simulink model "procestest"  (R2022b)
settings: Solver=VariableStepAuto  StartTime=0.0  StopTime=10.0  RelTol=1e-3
values from neighbouring files (symbols this model uses):
  A = 1/(4*tita*tita*sqrt(2))    [controllerId.m]    (also in identif_tf.m = 0.00679290871522)
  Cd = 1    [identif_tf.m]
  g = 9.8    [identif_tf.m]
  m = 2.7/1000    (= 0.0027)    [identif_tf.m]
  pwm_values = [0 20 60 100]    [identif_tf.m]
  q_points = [0 0.5 1.3 1.55]    [identif_tf.m]
  ro = 1.225    [identif_tf.m]
  Vb = (4*pi*(d_ball/2)^3)/3    (= 2.24492975038e-05)    [identif_tf.m]
settings Model: Creator=Admin  LastModifiedBy=Admin

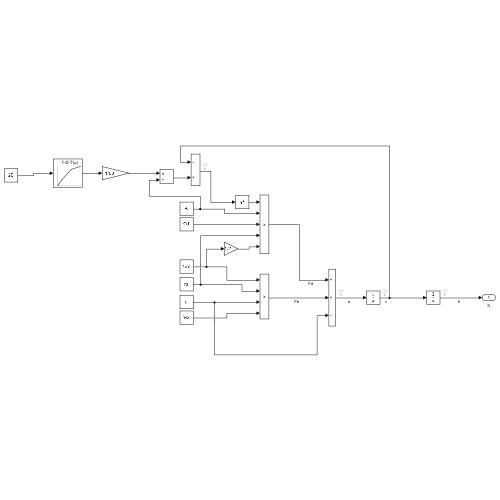
[thumbnail: Simulink's stored preview of the top-level diagram]
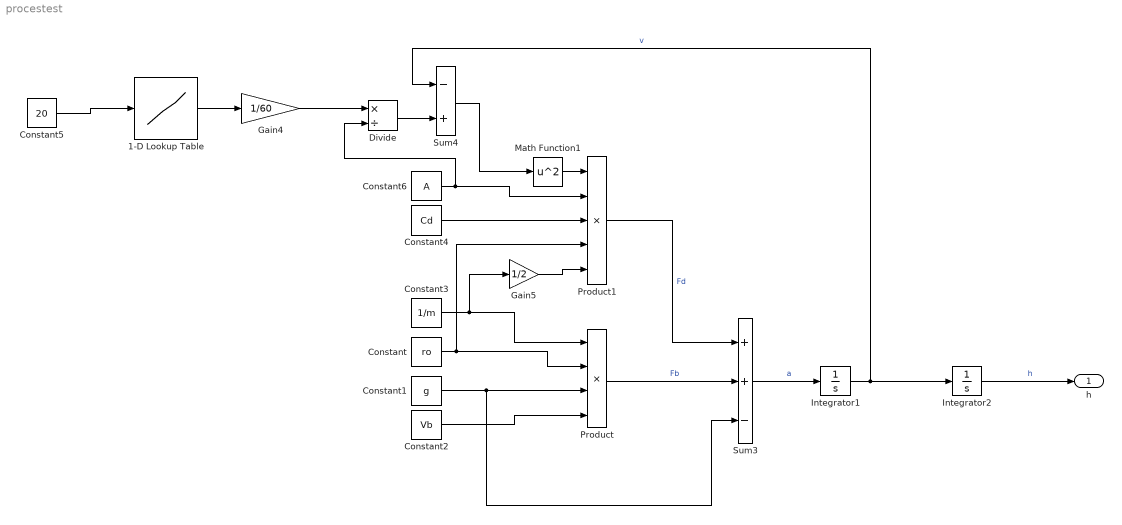
== system procestest ==
  1-D Lookup Table : Lookup_n-D  NumberOfTableDimensions=1  BreakpointsForDimension1=pwm_values  Table=q_points  InternalRulePriority=Speed  RndMeth=Simplest
  Constant : Constant  Value=ro
  Constant1 : Constant  Value=g
  Constant2 : Constant  Value=Vb
  Constant3 : Constant  Value=1/m
  Constant4 : Constant  Value=Cd
  Constant5 : Constant  Value=20
  Constant6 : Constant  Value=A
  Divide : Product  Inputs=*/
  Gain4 : Gain  Gain=1/60
  Gain5 : Gain  Gain=1/2
  Integrator1 : Integrator
  Integrator2 : Integrator
  Math Function1 : Math  Operator=square
  Product : Product  Inputs=4
  Product1 : Product  Inputs=5
  Sum3 : Sum  Inputs=++-
  Sum4 : Sum  Inputs=-+
  h : Outport
  wires:
  Divide/1 -> Sum4/2
  Sum4/1 -> Math Function1/1
  Product/1 -> Sum3/2  "Fb"
  Sum3/1 -> Integrator1/1  "a"
  Constant2/1 -> Product/4
  Gain4/1 -> Divide/1
  Constant1/1 -> Sum3/3, Product/3
  Constant4/1 -> Product1/3
  Constant5/1 -> 1-D Lookup Table/1
  Product1/1 -> Sum3/1  "Fd"
  Constant3/1 -> Gain5/1, Product/1
  1-D Lookup Table/1 -> Gain4/1
  Constant/1 -> Product1/4, Product/2
  Gain5/1 -> Product1/5
  Constant6/1 -> Divide/2, Product1/2
  Integrator2/1 -> h/1  "h"
  Math Function1/1 -> Product1/1
  Integrator1/1 -> Sum4/1, Integrator2/1  "v"
